simulink model "sm_excv_track2_ptcld_planar"  (R2026a)
settings: Solver=ode23t  StopTime=14  FixedStep=2e-4  AbsTol=1e-3
StartFcn:
  | tic
StopFcn:
  | Elapsed_Sim_Time = toc;
  | disp(['Elapsed Sim Time = ' num2str(Elapsed_Sim_Time)]);
undefined symbols (not defined in the file or in its folder): Excv, X, Y, Z
libraries: simulink x5, fl_lib x4, sm_lib x3, nesl_utility x3, sm_trackV_lib_terrain_contact_s46 x3, sm_excv_chassis_lib x2, sm_trackV_lib_chain_underc_elem x2, sm_trackV_lib_chain_lower_frame_s46i1u2l7 x2
CloseFcn:
  | try,close(h1_sm_excv_track_double),end
  | clear h1_sm_excv_track_double
  | try,close(h2_sm_excv_track_double),end
  | clear h2_sm_excv_track_double
  | try,close(h3_sm_excv_track_double),end
  | clear h3_sm_excv_track_double
  | try,close(h4_sm_excv_track_double),end
  | clear h4_sm_excv_track_double
  | 
  | 
  | clear simlog_sm_excv_track_double
  | clear logsout_sm_excv_track_double
Description:
  | Excavator Tracks (Planar), Ground Contact Point Cloud
  | Copyright 2023-2026 The MathWorks, Inc.
settings Model: Creator=evo  LastModifiedBy=smiller
settings SolverCC: ExtrapolationOrder=1.0
settings DataIOCC: SignalLoggingName=logsout_sm_excv_track2_ptcld_planar
settings DebuggingCC: SymbolicDimsDataTypeCodeGenerationDiagnostic=none
settings SimscapeCC: SimscapeNominalValues="[{\"value\":\"1\",\"unit\":\"A\"},{\"value\":\"1\",\"unit\":\"bar\"},{\"value\":\"1\",\"unit\":\"cm^2\"},{\"value\":\"1\",\"unit\":\"cm^3/s\"},{\"value\":\"1\",\"unit\":\"kJ/kg\"},{\"value\":\"1\",\"unit\":\"kW\"},{\"value\":\"1\",\"unit\":\"l\"},{\"value\":\"1\",\"unit\":\"N\"},{\"value\":\"1\",\"unit\":\"N*m\"},{\"value\":\"1\",\"unit\":\"V\"}]"  SimscapeLogSimulationStatistics=on  SimscapeLogName=simlog_sm_excv_track2_ptcld_planar  SimscapeLogLimitData=off
settings DiagnosticsConfigSet: SimMechanicsConflictingReferenceFrames=none
settings ExplorerConfigSet: InternalSimMechanicsExplorerSettings="<ExplorerConfiguration><canonicalview>default</canonicalview><AnimationSetting><BasePlaybackSpeed>1.0</BasePlaybackSpeed><PlaybackSpeedFactor>0.25</PlaybackSpeedFactor></AnimationSetting><TilePanel><TileInfo><Tiles Columns=\"2\" Count=\"3\" Rows=\"2\"><Column Weight=\"0.5\"/><Column Weight=\"0.5\"/><Row Weight=\"0.5\"/><Row Weight=\"0.5\"/><Tile Height=\"1\" Width=\"2\" X=\"0\" Y=\"0\"/><Tile Height=\"1\" Width=\"1\" X=\"0\" Y=\"1\"/><Tile Height=\"1\" Width=\"1\" X=\"1\" Y=\"1\"/></Tiles></TileInfo><SceneInfo><SceneViewer><BGColor><R>1</R><G>1</G><B>1</B></BGColor><Camera><DoPerspective>on</DoPerspective><Position><X>0</X><Y>-9.95285799552719998e-14</Y><Z>0.554946553288422351</Z></Position><Center><X>1</X><Y>-9.95285799552719998e-14</Y><Z>0.554946553288422351</Z></Center><Up><X>0</X><Y>0</Y><Z>1</Z></Up><ViewLimDist>1</ViewLimDist><YLim>0.466307658154998583</YLim><XLim>0.887968838401539839</XLim></Camera></SceneViewer><SceneViewer><BGColor><R>1</R><G>1</G><B>1</B></BGColor><Camera><DoPerspective>off</DoPerspective><Position><X>10.0004286080142499</X><Y>-63.1345143988139412</Y><Z>2.01677578846033079</Z></Position><Center><X>10.0000005340652702</X><Y>2.24533280857031059e-10</Y><Z>0.750000011139050793</Z></Center><Up><X>0.000675779963889239091</X><Y>0.0200606731361765434</Y><Z>0.999798536063523424</Z></Up><ViewLimDist>1</ViewLimDist><YLim>11.3757180156657967</YLim><XLim>10.6496083550913845</XLim></Camera></SceneViewer><SceneViewer><BGColor><R>1</R><G>1</G><B>1</B></BGColor><Camera><DoPerspective>on</DoPerspective><Position><X>1.68500000000005934</X><Y>-0.999999999999999556</Y><Z>0.554946553288429012</Z></Position><Center><X>1.68500000000000028</X><Y>4.44089209850062616e-16</Y><Z>0.554946553288422351</Z></Center><Up><X>0</X><Y>0</Y><Z>1</Z></Up><ViewLimDist>1</ViewLimDist><YLim>0.466307658154998583</YLim><XLim>0.436543339549360365</XLim></Camera></SceneViewer></SceneInfo></TilePanel><MechEditorPanel><Cameras><Camera><Id>Camera1</Id><Value><Name>Track_CtrRear_AimFront</Name><NativeCamera><PositionTrackingFeature>Chassis.Camera_Frames.CamF_CtrRear_AimLF.R</PositionTrackingFeature><CenterTrackingFeature>Config.World_Frame.W</CenterTrackingFeature><UpVectorTrackingFeature>Config.World_Frame.W</UpVectorTrackingFeature><CenterTrackingOrigin>off</CenterTrackingOrigin><CenterTrackingDirection>+X</CenterTrackingDirection><UpVectorTrackingDirection>+Z</UpVectorTrackingDirection></NativeCamera></Value></Camera><Camera><Id>Camera2</Id><Value><Name>Track_Left_AimRight</Name><NativeCamera><PositionTrackingFeature>Chassis.Camera_Frames.CamF_Left_AimRight.R</PositionTrackingFeature><CenterTrackingFeature>Chassis.Camera_Frames.CamF_Left_AimRight.R</CenterTrackingFeature><UpVectorTrackingFeature>Config.World_Frame.W</UpVectorTrackingFeature><CenterTrackingOrigin>off</CenterTrackingOrigin><CenterTrackingDirection>+X</CenterTrackingDirection><UpVectorTrackingDirection>+Z</UpVectorTrackingDirection></NativeCamera></Value></Camera><Camera><Id>Camera3</Id><Value><Name>Track_Front_AimLR</Name><NativeCamera><PositionTrackingFeature>Chassis.Camera_Frames.CamF_Front_AimLR.R</PositionTrackingFeature><CenterTrackingFeature>Chassis.Camera_Frames.Transform_Aim_LR.F</CenterTrackingFeature><UpVectorTrackingFeature>Config.World_Frame.W</UpVectorTrackingFeature><CenterTrackingOrigin>off</CenterTrackingOrigin><CenterTrackingDirection>+X</CenterTrackingDirection><UpVectorTrackingDirection>+Z</UpVectorTrackingDirection></NativeCamera></Value></Camera><Camera><Id>Camera4</Id><Value><Name>Track_Right_AimLeftTL</Name><NativeCamera><PositionTrackingFeature>Chassis.Camera_Frames.CamF_Right_AimLeftTL.R</PositionTrackingFeature><CenterTrackingFeature>Chassis.Camera_Frames.CamF_Right_AimLeftTL.R</CenterTrackingFeature><UpVectorTrackingFeature>Config.World_Frame.W</UpVectorTrackingFeature><CenterTrackingOrigin>off</CenterTrackingOrigin><CenterTrackingDirection>+X</CenterTrackingDirection><UpVectorTrackingDirection>+Z</UpVectorTrackingDirection></NativeCamera></Value></Camera><Camera><Id>Camera5</Id><Value><Name>Track_Right_AimLeftTR</Name><NativeCamera><PositionTrackingFeature>Chassis.Camera_Frames.CamF_Right_AimLeftTR.R</PositionTrackingFeature><CenterTrackingFeature>Chassis.Camera_Frames.CamF_Right_AimLeftTR.R</CenterTrackingFeature><UpVectorTrackingFeature>Config.World_Frame.W</UpVectorTrackingFeature><CenterTrackingOrigin>off</CenterTrackingOrigin><CenterTrackingDirection>+X</CenterTrackingDirection><UpVectorTrackingDirection>+Z</UpVectorTrackingDirection></NativeCamera></Value></Camera><Camera><Id>Camera6</Id><Value><Name>Track_FR_AimFront</Name><NativeCamera><PositionTrackingFeature>Chassis.Camera_Frames.CamF_FR_Aim_Front_R</PositionTrackingFeature><CenterTrackingFeature>Chassis.Camera_Frames.CamF_FR_Aim_Front_R</CenterTrackingFeature><UpVectorTrackingFeature>Config.W</UpVectorTrackingFeature><CenterTrackingOrigin>off</CenterTrackingOrigin><CenterTrackingDirection>+X</CenterTrackingDirection><UpVectorTrackingDirection>+Z</UpVectorTrackingDirection></NativeCamera></Value></Camera></Cameras><GfxPanelCameraMap><MapElement CameraMLId=\"Camera1\" GfxPanelIndex=\"0\"/><MapElement CameraMLId=\"Camera4\" GfxPanelIndex=\"2\"/></GfxPanelCameraMap><VideoCreator><PlaybackSpeedRatio>1.0</PlaybackSpeedRatio><FrameRate>30</FrameRate><VideoFormat>Motion JPEG AVI</VideoFormat><FrameSize>auto</FrameSize></VideoCreator></MechEditorPanel></ExplorerConfiguration>"

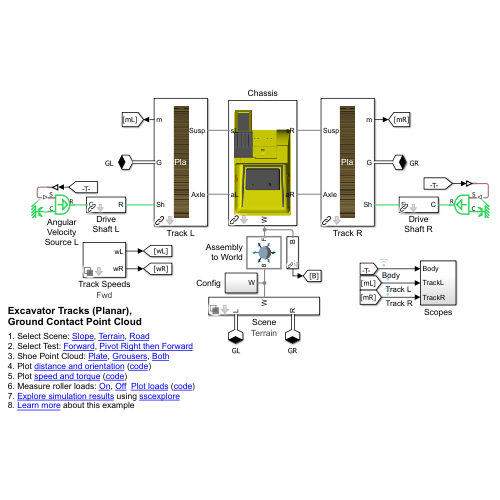
[thumbnail: Simulink's stored preview of the top-level diagram]
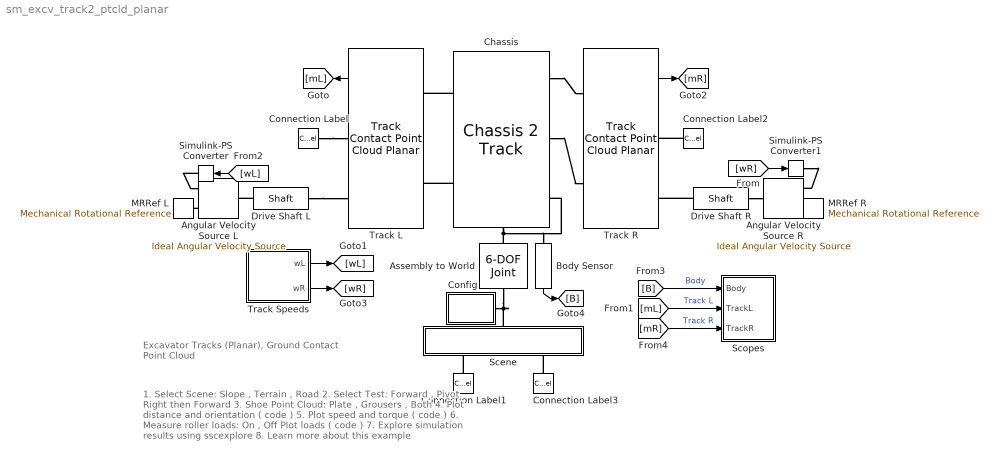
== system sm_excv_track2_ptcld_planar ==
  note: Excavator Tracks (Planar),
      | Ground Contact Point Cloud
  note: 1. Select Scene: Slope , Terrain , Road
      | 2. Select Test: Forward , Pivot Right then Forward
      | 3. Shoe Point Cloud: Plate , Grousers , Both
      | 4. Plot distance and orientation ( code )
      | 5. Plot speed and torque ( code )
      | 6. Measure roller loads: On , Off Plot loads ( code )
      | 7. Explore simulation results using sscexplore
      | 8. Learn more about this example
  Angular Velocity Source L : fl_lib/Mechanical/Mechanical Sources/Ideal Angular Velocity Source
  Angular Velocity Source R : fl_lib/Mechanical/Mechanical Sources/Ideal Angular Velocity Source
  Assembly to World : sm_lib/Joints/6-DOF Joint  JointMode=Normal  CompositeWrenchDir=FollowerOnBase  CompositeWrenchFrame=BaseFrame  SenseConstraintForce=off  SenseConstraintTorque=off  SenseTotalForce=off  SenseTotalTorque=off  PxPositionTargetSpecify=on  PxPositionTargetPriority=High  PxPositionTargetValue=0  PxPositionTargetValueUnits=m  PxVelocityTargetSpecify=off  PxVelocityTargetPriority=High  PxVelocityTargetValue=0  PxVelocityTargetValueUnits=m/s  PxEquilibriumPosition=0  PxEquilibriumPositionUnits=m  PxSpringStiffness=0  PxSpringStiffnessUnits=N/m  PxDampingCoefficient=0  PxDampingCoefficientUnits=N/(m/s)  PxLowerLimitSpecify=off  PxLowerLimitBound=-1  PxLowerLimitBoundUnits=m  PxLowerLimitStiffness=1e6  PxLowerLimitStiffnessUnits=N/m  PxLowerLimitDamping=1e3  PxLowerLimitDampingUnits=N/(m/s)  PxLowerLimitTransitionRegionWidth=1e-4  PxLowerLimitTransitionRegionWidthUnits=m  PxUpperLimitSpecify=off  PxUpperLimitBound=1  PxUpperLimitBoundUnits=m  PxUpperLimitStiffness=1e6  PxUpperLimitStiffnessUnits=N/m  PxUpperLimitDamping=1e3  PxUpperLimitDampingUnits=N/(m/s)  PxUpperLimitTransitionRegionWidth=1e-4  PxUpperLimitTransitionRegionWidthUnits=m  PxTorqueActuationMode=NoTorque  PxMotionActuationMode=ComputedMotion  PxSensePosition=off  PxSenseVelocity=off  PxSenseAcceleration=off  PxSenseTorqueForce=off  PxSenseLowerLimitTorqueForce=off  PxSenseUpperLimitTorqueForce=off  PyPositionTargetSpecify=on  PyPositionTargetPriority=High  PyPositionTargetValue=0  PyPositionTargetValueUnits=m  PyVelocityTargetSpecify=off  PyVelocityTargetPriority=High  PyVelocityTargetValue=0  PyVelocityTargetValueUnits=m/s  PyEquilibriumPosition=0  PyEquilibriumPositionUnits=m  PySpringStiffness=0  PySpringStiffnessUnits=N/m  PyDampingCoefficient=0  PyDampingCoefficientUnits=N/(m/s)  PyLowerLimitSpecify=off  PyLowerLimitBound=-1  PyLowerLimitBoundUnits=m  PyLowerLimitStiffness=1e6  PyLowerLimitStiffnessUnits=N/m  PyLowerLimitDamping=1e3  PyLowerLimitDampingUnits=N/(m/s)  PyLowerLimitTransitionRegionWidth=1e-4  PyLowerLimitTransitionRegionWidthUnits=m  PyUpperLimitSpecify=off  PyUpperLimitBound=1  PyUpperLimitBoundUnits=m  PyUpperLimitStiffness=1e6  PyUpperLimitStiffnessUnits=N/m  PyUpperLimitDamping=1e3  PyUpperLimitDampingUnits=N/(m/s)  PyUpperLimitTransitionRegionWidth=1e-4  PyUpperLimitTransitionRegionWidthUnits=m  PyTorqueActuationMode=NoTorque  PyMotionActuationMode=ComputedMotion  PySensePosition=off  PySenseVelocity=off  PySenseAcceleration=off  PySenseTorqueForce=off  PySenseLowerLimitTorqueForce=off  PySenseUpperLimitTorqueForce=off  PzPositionTargetSpecify=on  PzPositionTargetPriority=High  PzPositionTargetValue=Excv.Sprocket.sprocket_rPitch+0.2  PzPositionTargetValueUnits=m  PzVelocityTargetSpecify=off  PzVelocityTargetPriority=High  PzVelocityTargetValue=0  PzVelocityTargetValueUnits=m/s  PzEquilibriumPosition=0  PzEquilibriumPositionUnits=m  PzSpringStiffness=0  PzSpringStiffnessUnits=N/m  PzDampingCoefficient=0  PzDampingCoefficientUnits=N/(m/s)  PzLowerLimitSpecify=off  PzLowerLimitBound=-1  PzLowerLimitBoundUnits=m  PzLowerLimitStiffness=1e6  PzLowerLimitStiffnessUnits=N/m  PzLowerLimitDamping=1e3  PzLowerLimitDampingUnits=N/(m/s)  PzLowerLimitTransitionRegionWidth=1e-4  PzLowerLimitTransitionRegionWidthUnits=m  PzUpperLimitSpecify=off  PzUpperLimitBound=1  PzUpperLimitBoundUnits=m  PzUpperLimitStiffness=1e6  PzUpperLimitStiffnessUnits=N/m  PzUpperLimitDamping=1e3  PzUpperLimitDampingUnits=N/(m/s)  PzUpperLimitTransitionRegionWidth=1e-4  PzUpperLimitTransitionRegionWidthUnits=m  PzTorqueActuationMode=NoTorque  PzMotionActuationMode=ComputedMotion  PzSensePosition=off  PzSenseVelocity=off  PzSenseAcceleration=off  PzSenseTorqueForce=off  PzSenseLowerLimitTorqueForce=off  PzSenseUpperLimitTorqueForce=off  SphPositionTargetSpecify=off  SphPositionTargetPriority=High  SphPositionTargetRotationMethod=StandardAxis  SphPositionTargetFollAlignAxisA=+X  SphPositionTargetBaseAlignAxisA=+Y  SphPositionTargetFollAlignAxisB=+Y  SphPositionTargetBaseAlignAxisB=+Z  SphPositionTargetRotationStandardAxis=+Z  SphPositionTargetRotationAngle=180  SphPositionTargetRotationAngleUnits=deg  SphPositionTargetRotationArbitraryAxis=[0 0 1]  SphPositionTargetRotationSequenceAxes=FollowerAxes  SphPositionTargetRotationSequence=XYX  SphPositionTargetRotationSequenceAngles=[0 0 0]  SphPositionTargetRotationSequenceAnglesUnits=deg  SphPositionTargetRotationMatrix=[1 0 0; 0 1 0; 0 0 1]  SphPositionTargetQuaternion=[1 0 0 0]  SphVelocityTargetSpecify=off  SphVelocityTargetPriority=High  SphVelocityTargetValue=[0 0 0]  SphVelocityTargetValueUnits=deg/s  SphVelocityTargetInFollowerFrame=on  SphEqPosRotationMethod=None  SphEqPosFollAlignAxisA=+X  SphEqPosBaseAlignAxisA=+Y  SphEqPosFollAlignAxisB=+Y  SphEqPosBaseAlignAxisB=+Z  SphEqPosRotationStandardAxis=+Z  SphEqPosRotationAngle=0.0  SphEqPosRotationAngleUnits=deg  SphEqPosRotationArbitraryAxis=[0 0 1]  SphEqPosRotationSequenceAxes=FollowerAxes  SphEqPosRotationSequence=XYX  SphEqPosRotationSequenceAngles=[0 0 0]  SphEqPosRotationSequenceAnglesUnits=deg  SphEqPosRotationMatrix=[1 0 0; 0 1 0; 0 0 1]  SphEqPosQuaternion=[1 0 0 0]  SphSpringStiffness=0  SphSpringStiffnessUnits=N*m/deg  SphDampingCoefficient=0  SphDampingCoefficientUnits=N*m/(deg/s)  SphLowerLimitSpecify=off  SphLowerLimitBound=15  SphLowerLimitBoundUnits=deg  SphLowerLimitStiffness=1e4  SphLowerLimitStiffnessUnits=N*m/deg  SphLowerLimitDamping=10  SphLowerLimitDampingUnits=N*m/(deg/s)  SphLowerLimitTransitionRegionWidth=0.1  SphLowerLimitTransitionRegionWidthUnits=deg  SphUpperLimitSpecify=off  SphUpperLimitBound=45  SphUpperLimitBoundUnits=deg  SphUpperLimitStiffness=1e4  SphUpperLimitStiffnessUnits=N*m/deg  SphUpperLimitDamping=10  SphUpperLimitDampingUnits=N*m/(deg/s)  SphUpperLimitTransitionRegionWidth=0.1  SphUpperLimitTransitionRegionWidthUnits=deg  SphTorqueActuationMode=NoTorque  SphActuateTorqueX=off  SphActuateTorqueY=off  SphActuateTorqueZ=off  SphActuateTorque=off  SphActuationFrame=BaseFrame  SphSensePosition=off  SphSenseVelocityX=off  SphSenseVelocityY=off  SphSenseVelocityZ=off  SphSenseVelocity=off  SphSenseAccelerationX=off  SphSenseAccelerationY=off  SphSenseAccelerationZ=off  SphSenseAcceleration=off  SphSenseLowerLimitTorqueMag=off  SphSenseUpperLimitTorqueMag=off  SphSensingFrame=BaseFrame
  Body Sensor : sm_excv_chassis_lib/Body Sensor  offset_body_sensor=[0 0 0]
  Chassis : sm_excv_chassis_lib/Chassis 2 Track  offset_cg=Excv.Chassis.CGOffset  offset_axle=Excv.Chassis.AxleOffset  offset_Lcyl=Excv.Chassis.SuspOffset  offset_sprk2axle_x=Excv.Frame.AxleX  offset_sprk2axle_y=Excv.Frame.AxleY  Camera=Excv.Chassis.Camera  track_sep_ctr=Excv.Chassis.TrackSepCtr  axle_rad=Excv.Chassis.AxleRad  axle_opc=0  chassis_mass=Excv.Chassis.Mass  chassis_moi=Excv.Chassis.MOI  chassis_poi=Excv.Chassis.POI  body_clr=[1 1 0]  trim_clr=[0.4 0.4 0.4]  accent_clr=[1 0.6 0]  chassis_opc=1  cyl_len=Excv.Chassis.Susp.Cylinder.Cylinder.Len  cyl_rad=Excv.Chassis.Susp.Cylinder.Cylinder.Rad  cyl_mass=Excv.Chassis.Susp.Cylinder.Cylinder.Mass  piston_len=Excv.Chassis.Susp.Cylinder.Piston.Len  piston_rad=Excv.Chassis.Susp.Cylinder.Piston.Rad  piston_mass=Excv.Chassis.Susp.Cylinder.Piston.Mass  spr_k=Excv.Chassis.Susp.Cylinder.k  spr_d=Excv.Chassis.Susp.Cylinder.b  spr_xeq=Excv.Chassis.Susp.Cylinder.xeq
  Config : Subsystem
  Connection Label : ConnectionLabel  Label=GL
  Connection Label1 : ConnectionLabel  Label=GL
  Connection Label2 : ConnectionLabel  Label=GR
  Connection Label3 : ConnectionLabel  Label=GR
  Drive Shaft L : sm_trackV_lib_chain_underc_elem/Shaft  k_shaft=Excv.Drive.Shaft.k  b_shaft=Excv.Drive.Shaft.b
  Drive Shaft R : sm_trackV_lib_chain_underc_elem/Shaft  k_shaft=Excv.Drive.Shaft.k  b_shaft=Excv.Drive.Shaft.b
  MRRef L : fl_lib/Mechanical/Rotational Elements/Mechanical Rotational Reference
  MRRef R : fl_lib/Mechanical/Rotational Elements/Mechanical Rotational Reference
  Scene : Subsystem  Variant=on  VariantControlMode=label  LabelModeActiveChoice=Terrain
      settings: AttributesFormatString=%<LabelModeActiveChoice>
      mask Display: disp(' ');
  Scopes : Subsystem
  Simulink-PS Converter : nesl_utility/Simulink-PS Converter  PhysicalDomain=network_engine_domain  SubClassName=ps_input  LeftPortType=input  RightPortType=output  PseudoPeriodic=off  Frequencies=[]  NoiseDistribution=none  NoiseParameters=[]  Unit=1  AffineConversion=off  FilteringAndDerivatives=provide  SimscapeFilterOrder=1  InputFilterTimeConstant=0.001  UdotUserProvided=0
  Simulink-PS Converter1 : nesl_utility/Simulink-PS Converter  PhysicalDomain=network_engine_domain  SubClassName=ps_input  LeftPortType=input  RightPortType=output  PseudoPeriodic=off  Frequencies=[]  NoiseDistribution=none  NoiseParameters=[]  Unit=1  AffineConversion=off  FilteringAndDerivatives=provide  SimscapeFilterOrder=1  InputFilterTimeConstant=0.001  UdotUserProvided=0
  Track L : sm_trackV_lib_chain_lower_frame_s46i1u2l7/Track Contact Point Cloud Planar  popup_leftOrRight=Left  sprk_xc=Excv.Sprocket.sprocket_xc  sprk_len=Excv.Sprocket.sprk_width  sprk_rho=Excv.Sprocket.density  sprk_clr=Excv.Sprocket.clr  sprk_opc=Excv.Sprocket.opc  sprk_contact_geo_ptcld=Excv.Sprocket.teeth_contact.ptcld.pts(:,1:2)  sprk_contact_geo_rad=Excv.Sprocket.teeth_contact.ptcld.rad  sprk_contact_geo_clr=Excv.Sprocket.teeth_contact.ptcld.clr  sprk_contact_geo_opc=Excv.Sprocket.teeth_contact.ptcld.opc  idler_rad=Excv.Idler.rad  idler_len=Excv.Idler.len  idler_rho=Excv.Idler.rho  idler_clr=Excv.Idler.clr  idler_opc=Excv.Idler.opc  idler_contgeo_clr=Excv.Idler.chain_contact.clr  idler_contgeo_opc=Excv.Idler.chain_contact.opc  roller_upper_rad=Excv.Roller.Upper.rad  roller_upper_len=Excv.Roller.Upper.len  roller_upper_rho=Excv.Roller.Upper.rho  roller_upper_clr=Excv.Roller.Upper.clr  roller_upper_opc=Excv.Roller.Upper.opc  roller_upper_contgeo_clr=[1.0 0.0 0.0]  roller_upper_contgeo_opc=1  roller_lower_rad=Excv.Roller.Lower.rad  roller_lower_len=Excv.Roller.Lower.len  roller_lower_rho=Excv.Roller.Lower.rho  roller_lower_clr=Excv.Roller.Lower.clr  roller_lower_opc=Excv.Roller.Lower.opc  roller_lower_contgeo_clr=[1.0 0.0 0.0]  roller_lower_contgeo_opc=1  tensioner_cyl_len=Excv.Idler.Tensioner.cyl.len  tensioner_cyl_rad=Excv.Idler.Tensioner.cyl.rad  tensioner_cyl_rho=Excv.Idler.Tensioner.cyl.rho  tensioner_cyl_clr=Excv.Idler.Tensioner.cyl.clr  tensioner_cyl_opc=Excv.Idler.Tensioner.cyl.opc  tensioner_pist_len=Excv.Idler.Tensioner.piston.len  tensioner_pist_rad=Excv.Idler.Tensioner.piston.rad  tensioner_pist_rho=Excv.Idler.Tensioner.piston.rho  tensioner_pist_clr=Excv.Idler.Tensioner.piston.clr  tensioner_pist_opc=Excv.Idler.Tensioner.piston.opc  tensioner_br_length=Excv.Idler.Tensioner.bracket.len  tensioner_br_width=Excv.Idler.Tensioner.bracket.wid  tensioner_br_height=Excv.Idler.Tensioner.bracket.height  tensioner_br_thk=Excv.Idler.Tensioner.bracket.thk  tensioner_br_rho=Excv.Idler.Tensioner.bracket.rho  tensioner_br_clr=Excv.Idler.Tensioner.bracket.clr  tensioner_br_opc=Excv.Idler.Tensioner.bracket.opc  tensioner_eqpos=Excv.Idler.Tensioner.xeq  tensioner_x0=Excv.Idler.Tensioner.x0  tensioner_k=Excv.Idler.Tensioner.K  tensioner_b=Excv.Idler.Tensioner.B  roller_upper_x=Excv.Frame.Sprk2UpperX  roller_lower_x=Excv.Frame.Sprk2LowerX  idler_x=Excv.Frame.IdlerAssyX  axle_x=Excv.Frame.AxleX  roller_upper_y=Excv.Frame.Sprk2UpperY  roller_lower_y=Excv.Frame.Sprk2LowerY  idler_y=Excv.Frame.Sprk2IdlerY  axle_y=Excv.Frame.AxleY  sprk_pitch_rad=Excv.Sprocket.sprocket_rPitch  frame_cg_offset=Excv.Frame.CGOffset  frame_mass=Excv.Frame.Mass  frame_moi=Excv.Frame.MOI  frame_poi=Excv.Frame.POI  frame_susp_offset=Excv.Frame.SuspOffset  chain_wid=Excv.Chain.chain_wid  chain_seg_m=Excv.Chain.link_m  chain_seg_cg=Excv.Chain.link_cg  chain_seg_moi=Excv.Chain.link_moi  chain_seg_poi=Excv.Chain.link_poi  plate_xc=Excv.Chain.plate_xc  plate_h=Excv.Chain.plate_h  pin_sep=Excv.Chain.pin_sep  plate_thk=Excv.Chain.plate_thk  plate_ang=Excv.Chain.plate_ang  plate_clr=Excv.Chain.plate_clr  plate_opc=Excv.Chain.plate_opc  pin_len=Excv.Chain.pin_len  pin_rad=Excv.Chain.pin_rad  pin_clr=Excv.Chain.pin_clr  pin_opc=Excv.Chain.pin_opc  shoe_xc=Excv.Shoe.xc  shoe_w=Excv.Shoe.w  shoe_m=Excv.Shoe.mass  shoe_cg=Excv.Shoe.cg  shoe_moi=Excv.Shoe.moi  shoe_poi=Excv.Shoe.poi  shoe_clr=Excv.Shoe.clr  shoe_opc=Excv.Shoe.opc  jointTargets=track_joint_targets  chainDamping=Excv.Chain.damping  ptcld_shoe=Excv.Shoe.ground_contact.ptcld.pts  ptcld_shoe_rad=Excv.Shoe.ground_contact.ptcld.rad  ptcld_shoe_clr=Excv.Shoe.ground_contact.ptcld.clr  ptcld_shoe_opc=Excv.Shoe.ground_contact.ptcld.opc  chain_to_roller_clr=Excv.Chain.roller_contact.clr  chain_to_roller_opc=Excv.Chain.roller_contact.opc  chain_to_teeth_clr=Excv.Chain.teeth_contact.clr  chain_to_teeth_opc=Excv.Chain.teeth_contact.opc  B_Sprocket=Excv.Contact.Sprocket.B  K_Sprocket=Excv.Contact.Sprocket.K  TW_Sprocket=Excv.Contact.Sprocket.TW  K_Roller=Excv.Contact.Roller.K  B_Roller=Excv.Contact.Roller.B  TW_Roller=Excv.Contact.Roller.TW  K_Idler=Excv.Contact.Idler.K  B_Idler=Excv.Contact.Idler.B  TW_Idler=Excv.Contact.Idler.TW  popup_sense_roller=Actuator Torque
  Track R : sm_trackV_lib_chain_lower_frame_s46i1u2l7/Track Contact Point Cloud Planar  popup_leftOrRight=Right  sprk_xc=Excv.Sprocket.sprocket_xc  sprk_len=Excv.Sprocket.sprk_width  sprk_rho=Excv.Sprocket.density  sprk_clr=Excv.Sprocket.clr  sprk_opc=Excv.Sprocket.opc  sprk_contact_geo_ptcld=Excv.Sprocket.teeth_contact.ptcld.pts(:,1:2)  sprk_contact_geo_rad=Excv.Sprocket.teeth_contact.ptcld.rad  sprk_contact_geo_clr=Excv.Sprocket.teeth_contact.ptcld.clr  sprk_contact_geo_opc=Excv.Sprocket.teeth_contact.ptcld.opc  idler_rad=Excv.Idler.rad  idler_len=Excv.Idler.len  idler_rho=Excv.Idler.rho  idler_clr=Excv.Idler.clr  idler_opc=Excv.Idler.opc  idler_contgeo_clr=Excv.Idler.chain_contact.clr  idler_contgeo_opc=Excv.Idler.chain_contact.opc  roller_upper_rad=Excv.Roller.Upper.rad  roller_upper_len=Excv.Roller.Upper.len  roller_upper_rho=Excv.Roller.Upper.rho  roller_upper_clr=Excv.Roller.Upper.clr  roller_upper_opc=Excv.Roller.Upper.opc  roller_upper_contgeo_clr=[1.0 0.0 0.0]  roller_upper_contgeo_opc=1  roller_lower_rad=Excv.Roller.Lower.rad  roller_lower_len=Excv.Roller.Lower.len  roller_lower_rho=Excv.Roller.Lower.rho  roller_lower_clr=Excv.Roller.Lower.clr  roller_lower_opc=Excv.Roller.Lower.opc  roller_lower_contgeo_clr=[1.0 0.0 0.0]  roller_lower_contgeo_opc=1  tensioner_cyl_len=Excv.Idler.Tensioner.cyl.len  tensioner_cyl_rad=Excv.Idler.Tensioner.cyl.rad  tensioner_cyl_rho=Excv.Idler.Tensioner.cyl.rho  tensioner_cyl_clr=Excv.Idler.Tensioner.cyl.clr  tensioner_cyl_opc=Excv.Idler.Tensioner.cyl.opc  tensioner_pist_len=Excv.Idler.Tensioner.piston.len  tensioner_pist_rad=Excv.Idler.Tensioner.piston.rad  tensioner_pist_rho=Excv.Idler.Tensioner.piston.rho  tensioner_pist_clr=Excv.Idler.Tensioner.piston.clr  tensioner_pist_opc=Excv.Idler.Tensioner.piston.opc  tensioner_br_length=Excv.Idler.Tensioner.bracket.len  tensioner_br_width=Excv.Idler.Tensioner.bracket.wid  tensioner_br_height=Excv.Idler.Tensioner.bracket.height  tensioner_br_thk=Excv.Idler.Tensioner.bracket.thk  tensioner_br_rho=Excv.Idler.Tensioner.bracket.rho  tensioner_br_clr=Excv.Idler.Tensioner.bracket.clr  tensioner_br_opc=Excv.Idler.Tensioner.bracket.opc  tensioner_eqpos=Excv.Idler.Tensioner.xeq  tensioner_x0=Excv.Idler.Tensioner.x0  tensioner_k=Excv.Idler.Tensioner.K  tensioner_b=Excv.Idler.Tensioner.B  roller_upper_x=Excv.Frame.Sprk2UpperX  roller_lower_x=Excv.Frame.Sprk2LowerX  idler_x=Excv.Frame.IdlerAssyX  axle_x=Excv.Frame.AxleX  roller_upper_y=Excv.Frame.Sprk2UpperY  roller_lower_y=Excv.Frame.Sprk2LowerY  idler_y=Excv.Frame.Sprk2IdlerY  axle_y=Excv.Frame.AxleY  sprk_pitch_rad=Excv.Sprocket.sprocket_rPitch  frame_cg_offset=Excv.Frame.CGOffset  frame_mass=Excv.Frame.Mass  frame_moi=Excv.Frame.MOI  frame_poi=Excv.Frame.POI  frame_susp_offset=Excv.Frame.SuspOffset  chain_wid=Excv.Chain.chain_wid  chain_seg_m=Excv.Chain.link_m  chain_seg_cg=Excv.Chain.link_cg  chain_seg_moi=Excv.Chain.link_moi  chain_seg_poi=Excv.Chain.link_poi  plate_xc=Excv.Chain.plate_xc  plate_h=Excv.Chain.plate_h  pin_sep=Excv.Chain.pin_sep  plate_thk=Excv.Chain.plate_thk  plate_ang=Excv.Chain.plate_ang  plate_clr=Excv.Chain.plate_clr  plate_opc=Excv.Chain.plate_opc  pin_len=Excv.Chain.pin_len  pin_rad=Excv.Chain.pin_rad  pin_clr=Excv.Chain.pin_clr  pin_opc=Excv.Chain.pin_opc  shoe_xc=Excv.Shoe.xc  shoe_w=Excv.Shoe.w  shoe_m=Excv.Shoe.mass  shoe_cg=Excv.Shoe.cg  shoe_moi=Excv.Shoe.moi  shoe_poi=Excv.Shoe.poi  shoe_clr=Excv.Shoe.clr  shoe_opc=Excv.Shoe.opc  jointTargets=track_joint_targets  chainDamping=Excv.Chain.damping  ptcld_shoe=Excv.Shoe.ground_contact.ptcld.pts  ptcld_shoe_rad=Excv.Shoe.ground_contact.ptcld.rad  ptcld_shoe_clr=Excv.Shoe.ground_contact.ptcld.clr  ptcld_shoe_opc=Excv.Shoe.ground_contact.ptcld.opc  chain_to_roller_clr=Excv.Chain.roller_contact.clr  chain_to_roller_opc=Excv.Chain.roller_contact.opc  chain_to_teeth_clr=Excv.Chain.teeth_contact.clr  chain_to_teeth_opc=Excv.Chain.teeth_contact.opc  B_Sprocket=Excv.Contact.Sprocket.B  K_Sprocket=Excv.Contact.Sprocket.K  TW_Sprocket=Excv.Contact.Sprocket.TW  K_Roller=Excv.Contact.Roller.K  B_Roller=Excv.Contact.Roller.B  TW_Roller=Excv.Contact.Roller.TW  K_Idler=Excv.Contact.Idler.K  B_Idler=Excv.Contact.Idler.B  TW_Idler=Excv.Contact.Idler.TW  popup_sense_roller=Actuator Torque
  Track Speeds : Subsystem  Variant=on  VariantControlMode=label  VariantControl=Choice  LabelModeActiveChoice=Fwd
      settings: AttributesFormatString=%<LabelModeActiveChoice>
      mask Display: disp(' ')
  wires:
  Track L/1 -> [mL]
  [mL] -> Scopes/2(TrackL)  "Track L"
  Track R/1 -> [mR]
  [mR] -> Scopes/3(TrackR)  "Track R"
  Track Speeds/1(wL) -> [wL]
  [wL] -> Simulink-PS Converter/1
  Track Speeds/2(wR) -> [wR]
  [wR] -> Simulink-PS Converter1/1
  Body Sensor/1 -> [B]
  [B] -> Scopes/1(Body)  "Body"
  connections:
  Assembly to World/LConn1 -- Scene/RConn1 -- Config/LConn1
  Assembly to World/RConn1 -- Body Sensor/LConn1 -- Chassis/RConn3
  Drive Shaft L/LConn1 -- Angular Velocity Source L/LConn1
  Simulink-PS Converter/RConn1 -- Angular Velocity Source L/RConn1
  Angular Velocity Source L/RConn2 -- MRRef L/LConn1
  Angular Velocity Source R/RConn2 -- MRRef R/LConn1
  Simulink-PS Converter1/RConn1 -- Angular Velocity Source R/RConn1
  Drive Shaft R/LConn1 -- Angular Velocity Source R/LConn1
  Chassis/LConn1 -- Track L/LConn1
  Chassis/LConn2 -- Track L/LConn2
  Chassis/RConn2 -- Track R/LConn2
  Chassis/RConn1 -- Track R/LConn1
  Drive Shaft R/RConn1 -- Track R/RConn2
  Drive Shaft L/RConn1 -- Track L/RConn2
  Connection Label/LConn1 -- Track L/RConn1
  Connection Label2/LConn1 -- Track R/RConn1
  Connection Label3/LConn1 -- Scene/LConn2
  Connection Label1/LConn1 -- Scene/LConn1

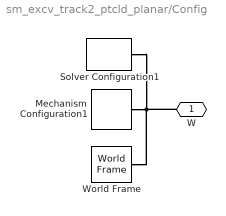
== system sm_excv_track2_ptcld_planar/Config ==
  Mechanism Configuration1 : sm_lib/Utilities/Mechanism Configuration  UniformGravity=Constant  GravityVector=[0 0 -9.80665]  GravityVectorUnits=m/s^2  LinearizationDelta=0.001  JointModeTransitionNonlinearIterations=2
  Solver Configuration1 : nesl_utility/Solver Configuration  PhysicalDomain=network_engine_domain  SubClassName=solver  LeftPortType=input  RightPortType=generic  Tones=[]  Harmonics=[]  SimulateNoise=off  Profile=off  UseLocalSampling=off  EnableSwitchedLinearOptims=on  FrequencyDomain=off  UseCCode=off  RelTol=0.001  AbsTol=0.001  MinStep=1e-09  ToWorkspace=off  RevertToSquareIcSolve=off  NumHomotopyIterations=100  PhasorMode=off  PhasorModeNumHarmonics=1  ConsistencySolver=NEWTON_FTOL  CanonicalOrdering=UNORDERED  OptimizeIntermediates=UNOPTIMIZED  IndexReductionMethod=DerivativeReplacement  DoDC=off  ResidualTolerance=1e-09  ConsistencyTolSource=GLOBAL  ConsistencyAbsTol=0.001  ConsistencyRelTol=0.001  ConsistencyTolFactor=0.001  UseLocalSolver=off  LocalSolverChoice=NE_BACKWARD_EULER_ADVANCER  ResolveIndetEquations=on  FunctionEvalNumThread=1  LocalSolverSampleTime=0.001  DoFixedCost=off  MaxNonlinIter=3  MaxModeIter=2  ComputeImpulses=off  ImpulseIterations=2  LinearAlgebra=auto  LinearAlgebraNumThread=0  EquationFormulation=NE_TIME_EF  DelaysMemoryBudget=1024  AutomaticFiltering=on  FilteringTimeConstant=0.001  PartitionStorageMethod=AS_NEEDED  PartitionMemoryBudget=1024  PartitionMethod=ROBUST  MultibodyUseLocalSolver=off  MultibodyLocalSolverChoice=ODE1  MultibodyLocalSolverSampleTime=0.001
  World Frame : sm_lib/Frames and Transforms/World Frame
  W : PMIOPort  Side=Left
  connections:
  W/RConn1 -- Solver Configuration1/RConn1 -- Mechanism Configuration1/RConn1 -- World Frame/RConn1

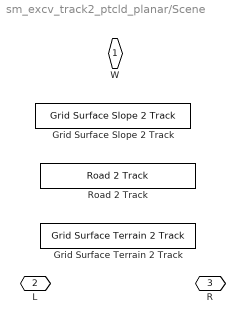
== system sm_excv_track2_ptcld_planar/Scene ==
  Grid Surface Slope 2 Track : sm_trackV_lib_terrain_contact_s46/Grid Surface Slope 2 Track  VariantControl=Slope  road_len=Scene.Slope.road_len  road_wid=Scene.Slope.road_wid  slope_rise=Scene.Slope.slope_rise  slope_run=Scene.Slope.slope_run  slope_x0=Scene.Slope.slope_start  slope_xres=Scene.Slope.slope_xres  surface_clr=Scene.Slope.clr  surface_opc=Scene.Slope.opc  TW_Road=Scene.Contact.Terrain.TW  B_Road=Scene.Contact.Terrain.B  K_Road=Scene.Contact.Terrain.K  F_dyn_Road=Scene.Contact.Terrain.mud  F_stat_Road=Scene.Contact.Terrain.mus  CV_Road=Scene.Contact.Terrain.CV
  Grid Surface Terrain 2 Track : sm_trackV_lib_terrain_contact_s46/Grid Surface Terrain 2 Track  SystemSampleTime=-1  VariantControl=Terrain  VariantActivationTime=update diagram  EmptyChoice=off  PassThrough=off  PassThroughVariantControl=(default)  EmptyChoiceVariantControl=(default)  AllowFlexibleInterface=on  Latency=0  AutoFrameSizeCalculation=off
  Road 2 Track : sm_trackV_lib_terrain_contact_s46/Road 2 Track  SystemSampleTime=-1  VariantControl=Road  VariantActivationTime=update diagram  EmptyChoice=off  PassThrough=off  PassThroughVariantControl=(default)  EmptyChoiceVariantControl=(default)  AllowFlexibleInterface=on  Latency=0  AutoFrameSizeCalculation=off
  W : PMIOPort  Side=Right
  L : PMIOPort  Port=2  Side=Left
  R : PMIOPort  Port=3  Side=Left

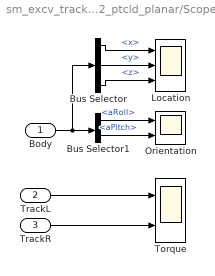
== system sm_excv_track2_ptcld_planar/Scopes ==
  Body : Inport
  TrackL : Inport  Port=2
  TrackR : Inport  Port=3
  Bus Selector : BusSelector  OutputSignals=x,y,z
  Bus Selector1 : BusSelector  OutputSignals=aRoll,aPitch
  Location : Scope  NumInputPorts=3
      settings: ActiveDisplayYMinimum=-2.438  ActiveDisplayYMaximum=13.72233
  Orientation : Scope  NumInputPorts=2
      settings: ActiveDisplayYMinimum=-0.40552  ActiveDisplayYMaximum=0.36121  DataLoggingVariableName=ScopeData2
  Torque : Scope  NumInputPorts=2
  wires:
  Body/1 -> Bus Selector/1, Bus Selector1/1
  Bus Selector/3 -> Location/3  "<z>"
  TrackL/1 -> Torque/1
  Bus Selector1/1 -> Orientation/1  "<aRoll>"
  Bus Selector/2 -> Location/2  "<y>"
  Bus Selector/1 -> Location/1  "<x>"
  Bus Selector1/2 -> Orientation/2  "<aPitch>"
  TrackR/1 -> Torque/2

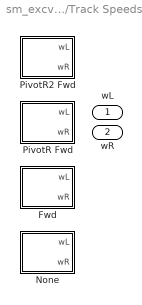
== system sm_excv_track2_ptcld_planar/Track Speeds ==
  Fwd : Subsystem  VariantControl=Fwd
  None : Subsystem  VariantControl=None
  PivotR Fwd : Subsystem  VariantControl=PivotR_Fwd
  PivotR2 Fwd : Subsystem  VariantControl=PivotR2_Fwd
  wL : Outport
  wR : Outport  Port=2

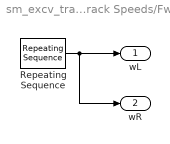
== system sm_excv_track2_ptcld_planar/Track Speeds/Fwd ==
  Repeating Sequence : simulink/Sources/Repeating Sequence  rep_seq_t=[0 2 2.01 40]  rep_seq_y=[0 0 3 3]
  wL : Outport
  wR : Outport  Port=2
  wires:
  Repeating Sequence/1 -> wR/1, wL/1

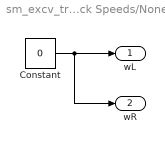
== system sm_excv_track2_ptcld_planar/Track Speeds/None ==
  Constant : Constant  Value=0
  wL : Outport
  wR : Outport  Port=2
  wires:
  Constant/1 -> wL/1, wR/1

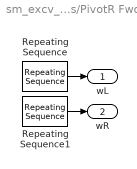
== system sm_excv_track2_ptcld_planar/Track Speeds/PivotR Fwd ==
  Repeating Sequence : simulink/Sources/Repeating Sequence  rep_seq_t=[0 2 2.01 40]  rep_seq_y=[0 0 3 3]
  Repeating Sequence1 : simulink/Sources/Repeating Sequence  rep_seq_t=[0 2 2.01 2.5 2.51 40]  rep_seq_y=[0 0 -3 -3 3 3]
  wL : Outport
  wR : Outport  Port=2
  wires:
  Repeating Sequence1/1 -> wR/1
  Repeating Sequence/1 -> wL/1

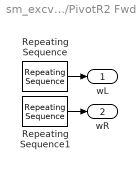
== system sm_excv_track2_ptcld_planar/Track Speeds/PivotR2 Fwd ==
  Repeating Sequence : simulink/Sources/Repeating Sequence  rep_seq_t=[0 2 2.01 40]  rep_seq_y=[0 0 3 3]
  Repeating Sequence1 : simulink/Sources/Repeating Sequence  rep_seq_t=[0 2 2.01 5.5 5.51 40]  rep_seq_y=[0 0 -3 -3 3 3]
  wL : Outport
  wR : Outport  Port=2
  wires:
  Repeating Sequence/1 -> wL/1
  Repeating Sequence1/1 -> wR/1
